simulink model "ball_simulation"  (R2019a)
settings: Solver=FixedStepAuto  StartTime=0.0  StopTime=5  FixedStep=0.001  RelTol=1e-3
values from neighbouring files (symbols this model uses):
  g = 9.8    [ball_control.m]
  K_tot = blkdiag (K_pd, K_pd, K_pd)    [ball_control.m]
  mass = 0.01    [ball_control.m]
  Nx = blkdiag ([1; 0], [1; 0], [1; 0])    [ball_control.m]
  reorder_mx = [E(:,1), E(:,3), E(:,5), E(:,2), E(:,4), E(:,6)]    [ball_control.m]
settings Model: Creator=nicola  LastModifiedBy=nicola

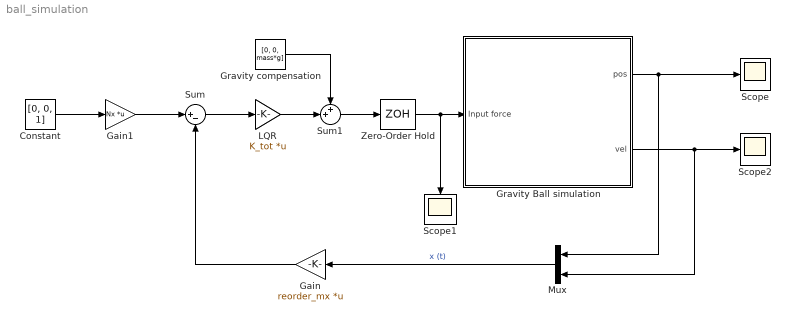
== system ball_simulation ==
  Constant : Constant  Value=[0, 0, 1]
  Gain : Gain  Gain=reorder_mx  Multiplication=Matrix(K*u)
  Gain1 : Gain  Gain=Nx  Multiplication=Matrix(K*u)
  Gravity Ball simulation : Subsystem
  Gravity compensation : Constant  Value=[0, 0, mass*g]
  LQR : Gain  Gain=K_tot  Multiplication=Matrix(K*u)
  Mux : Mux  Inputs=2
  Scope : Scope
  Scope1 : Scope
  Scope2 : Scope
  Sum : Sum  Inputs=|+-
  Sum1 : Sum  Inputs=++|
  Zero-Order Hold : ZeroOrderHold  SampleTime=0.02
  wires:
  Gravity Ball simulation/1(pos) -> Mux/1, Scope/1
  Gravity Ball simulation/2(vel) -> Mux/2, Scope2/1
  Constant/1 -> Gain1/1
  Sum/1 -> LQR/1
  Mux/1 -> Gain/1  "x (t)"
  Sum1/1 -> Zero-Order Hold/1
  Gravity compensation/1 -> Sum1/1
  LQR/1 -> Sum1/2
  Gain1/1 -> Sum/1
  Gain/1 -> Sum/2
  Zero-Order Hold/1 -> Scope1/1, Gravity Ball simulation/1(Input force)

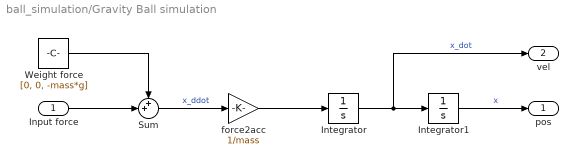
== system ball_simulation/Gravity Ball simulation ==
  Input force : Inport
  Integrator : Integrator  InitialCondition=[0, 0, 0]
  Integrator1 : Integrator  InitialCondition=[0, 0, 0]
  Sum : Sum  Inputs=++|
  Weight force : Constant  Value=[0, 0, -mass*g]
  force2acc : Gain  Gain=1/mass
  pos : Outport
  vel : Outport  Port=2
  wires:
  Weight force/1 -> Sum/1
  Integrator1/1 -> pos/1  "x"
  Input force/1 -> Sum/2
  Sum/1 -> force2acc/1  "x_ddot"
  Integrator/1 -> vel/1, Integrator1/1  "x_dot"
  force2acc/1 -> Integrator/1
